simulink model "Project_Earth_Pointing"  (R2022b)
settings: Solver=VariableStepAuto  StartTime=0.0  StopTime=1000  RelTol=1e-3
values from neighbouring files (symbols this model uses):
  a = (Rp+Ra)/2    [trial_complete_project.m]    (also in trial_detumbling.m; trial_earth_pointing.m)
  A0 = Ax*Ay*Az    [trial_complete_project.m]    (also in trial_detumbling.m = [0.5391 0.1008 0.8362; -0.3591 0.9255 0.1200; -0.7618 -0.365; trial_earth_pointing.m = [-0.2505 -0.7848 0.5668; 0.7978 0.1644 0.5801; -0.5485 0.597)
  A1 = L1*L2    (= 0.06)    [trial_complete_project.m]    (also in trial_detumbling.m; trial_earth_pointing.m)
  A10 = A1    (= 0.06)    [trial_complete_project.m]    (also in trial_detumbling.m; trial_earth_pointing.m)
  A2 = A1    (= 0.06)    [trial_complete_project.m]    (also in trial_detumbling.m; trial_earth_pointing.m)
  A3 = L1*L3    (= 0.03)    [trial_complete_project.m]    (also in trial_detumbling.m; trial_earth_pointing.m)
  A4 = A3    (= 0.03)    [trial_complete_project.m]    (also in trial_detumbling.m; trial_earth_pointing.m)
  A5 = L2*L3    (= 0.02)    [trial_complete_project.m]    (also in trial_detumbling.m; trial_earth_pointing.m)
  A6 = A5    (= 0.02)    [trial_complete_project.m]    (also in trial_detumbling.m; trial_earth_pointing.m)
  A7 = A1    (= 0.06)    [trial_complete_project.m]    (also in trial_detumbling.m; trial_earth_pointing.m)
  A8 = A1    (= 0.06)    [trial_complete_project.m]    (also in trial_detumbling.m; trial_earth_pointing.m)
  A9 = A1    (= 0.06)    [trial_complete_project.m]    (also in trial_detumbling.m; trial_earth_pointing.m)
  a_s = 149600000    [trial_complete_project.m]    (also in trial_detumbling.m; trial_earth_pointing.m)
  alpha1 = 0.9    [trial_complete_project.m]    (also in trial_detumbling.m; trial_earth_pointing.m)
  alpha2 = 0.1    [trial_complete_project.m]    (also in trial_detumbling.m; trial_earth_pointing.m)
  alphaState_obs = -0.9    [trial_complete_project.m]    (also in trial_detumbling.m; trial_earth_pointing.m)
  an = (11.5*pi)/180    (= 0.200712863979)    [trial_complete_project.m]    (also in trial_detumbling.m; trial_earth_pointing.m)
  e = (Ra-Rp)/(Ra+Rp)    [trial_complete_project.m]    (also in trial_detumbling.m; trial_earth_pointing.m)
  e_s = 0.0167086    [trial_complete_project.m]    (also in trial_detumbling.m; trial_earth_pointing.m)
  i = 0*pi/180    (= 0)    [trial_complete_project.m]    (also in trial_detumbling.m; trial_earth_pointing.m)
  I_x = 0.059029338    [trial_complete_project.m]    (also in trial_detumbling.m; trial_earth_pointing.m = 0.093296)
  I_y = 0.116709338    [trial_complete_project.m]    (also in trial_detumbling.m; trial_earth_pointing.m = 0.161261916)
  I_z = 0.149968    [trial_complete_project.m]    (also in trial_detumbling.m; trial_earth_pointing.m = 0.160253916)
  kdx = kd*(I_x/I)    (= 1.44987726319)    [trial_complete_project.m]    (also in trial_detumbling.m; trial_earth_pointing.m = 2.6989394073)
  kdy = kd*(I_y/I)    (= 2.86661211697)    [trial_complete_project.m]    (also in trial_detumbling.m; trial_earth_pointing.m = 4.66511040119)
  kdz = kd*(I_z/I)    (= 3.68351061984)    [trial_complete_project.m]    (also in trial_detumbling.m; trial_earth_pointing.m = 4.63595019151)
  kpx = kp*(I_x/I)    (= 0.0163111192108)    [trial_complete_project.m]    (also in trial_detumbling.m; trial_earth_pointing.m = 0.0202420455548)
  kpy = kp*(I_y/I)    (= 0.0322493863159)    [trial_complete_project.m]    (also in trial_detumbling.m; trial_earth_pointing.m = 0.0349883280089)
  kpz = kp*(I_z/I)    (= 0.0414394944732)    [trial_complete_project.m]    (also in trial_detumbling.m; trial_earth_pointing.m = 0.0347696264363)
  kState_obs = 0.9    [trial_complete_project.m]    (also in trial_detumbling.m; trial_earth_pointing.m)
  m = [0.01 0.05 0.01]    [trial_complete_project.m]    (also in trial_detumbling.m; trial_earth_pointing.m)
  mu = astroConstants(13)    [trial_complete_project.m]    (also in trial_detumbling.m; trial_earth_pointing.m)
  n = sqrt(mu/a^3)    [trial_complete_project.m]    (also in trial_detumbling.m; trial_earth_pointing.m)
  n_s = sqrt(mu_s/a_s^3)    [trial_complete_project.m]    (also in trial_detumbling.m; trial_earth_pointing.m)
  P = F_e/c    (= 4.52980041279e-06)    [trial_complete_project.m]    (also in trial_detumbling.m; trial_earth_pointing.m)
  P_E = F_earth/c    (= 2.23487943783e-06)    [trial_complete_project.m]    (also in trial_detumbling.m; trial_earth_pointing.m)
  pd_sc = 0.1    [trial_complete_project.m]    (also in trial_detumbling.m; trial_earth_pointing.m)
  pd_sp = 0.1    [trial_complete_project.m]    (also in trial_detumbling.m; trial_earth_pointing.m)
  ps_sc = 0.5    [trial_complete_project.m]    (also in trial_detumbling.m; trial_earth_pointing.m)
  ps_sp = 0.1    [trial_complete_project.m]    (also in trial_detumbling.m; trial_earth_pointing.m)
  r = astroConstants(23)    [trial_complete_project.m]    (also in trial_detumbling.m; trial_earth_pointing.m)
  r1 = [0;0;-L3/2] + c_m    [trial_complete_project.m]    (also in trial_detumbling.m; trial_earth_pointing.m)
  r10 = r9    [trial_complete_project.m]    (also in trial_detumbling.m; trial_earth_pointing.m)
  r2 = [0; 0 ;L3/2] + c_m    [trial_complete_project.m]    (also in trial_detumbling.m; trial_earth_pointing.m)
  r3 = [0; L2/2;0] + c_m    [trial_complete_project.m]    (also in trial_detumbling.m; trial_earth_pointing.m)
  r4 = [0; -L2/2;0] + c_m    [trial_complete_project.m]    (also in trial_detumbling.m; trial_earth_pointing.m)
  r5 = [-L1/2; 0 ;0] + c_m    [trial_complete_project.m]    (also in trial_detumbling.m; trial_earth_pointing.m)
  r6 = [L1/2; 0;0]+ c_m    [trial_complete_project.m]    (also in trial_detumbling.m; trial_earth_pointing.m)
  r7 = [-L1/2; 0 ; L3/2 + L1/2] + c_m    [trial_complete_project.m]    (also in trial_detumbling.m; trial_earth_pointing.m)
  r8 = r7    [trial_complete_project.m]    (also in trial_detumbling.m; trial_earth_pointing.m)
  r9 = [-L1/2; 0 ; -L3/2 - L1/2]    [trial_complete_project.m]    (also in trial_detumbling.m; trial_earth_pointing.m)
  RW = 0.002    [trial_complete_project.m]    (also in trial_detumbling.m; trial_earth_pointing.m)
  theta0 = 0    [trial_complete_project.m]    (also in trial_detumbling.m; trial_earth_pointing.m)
  w0_x = 1    [trial_complete_project.m]    (also in trial_detumbling.m; trial_earth_pointing.m = -0.008328)
  w0_y = 1    [trial_complete_project.m]    (also in trial_detumbling.m; trial_earth_pointing.m = 0.004962)
  w0_z = 1    [trial_complete_project.m]    (also in trial_detumbling.m; trial_earth_pointing.m = -0.0004756)
  w_E = (15.04*pi/180)/3600    (= 7.29159776389e-05)    [trial_complete_project.m]    (also in trial_detumbling.m; trial_earth_pointing.m)
libraries: matrix_library x28, vrlib x7, dspinverses x1
(part 1 of 3)
settings Model: Creator=PEPPE  LastModifiedBy=PEPPE
settings SolverCC: ZeroCrossAlgorithm=Adaptive
settings DebuggingCC: IgnoredZcDiagnostic=none

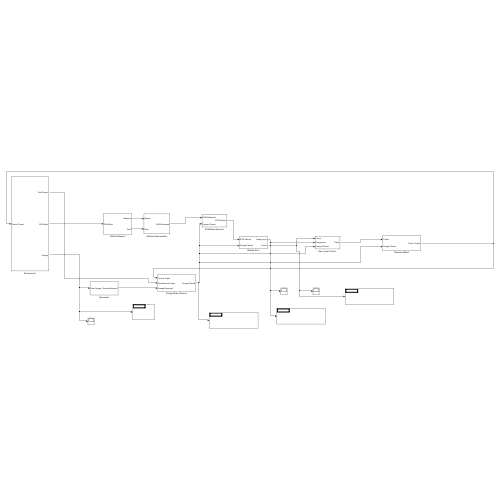
[thumbnail: Simulink's stored preview of the top-level diagram]
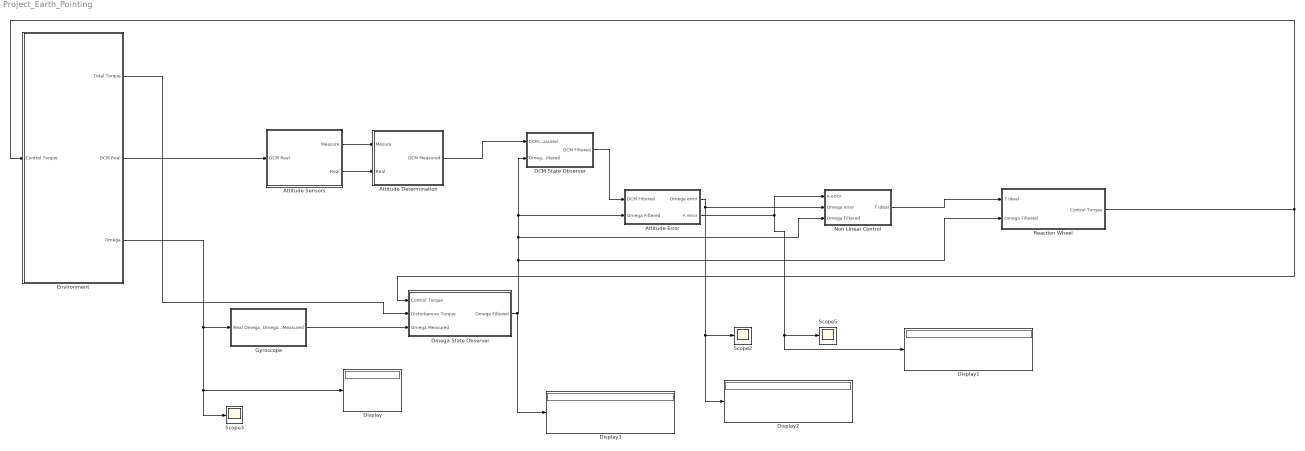
== system Project_Earth_Pointing ==
  Attitude Determination : Subsystem
  Attitude Error : Subsystem
  Attitude Sensors : Subsystem
  DCM State Observer : Subsystem
  Display{,1..3} (4 alike) : Display
  Environment : Subsystem
  Gyroscope : Subsystem
  "Non Linear Control " : Subsystem
  Omega State Observer : Subsystem
  Reaction Wheel : Subsystem
  Scope2 : Scope
  Scope3 : Scope
  Scope5 : Scope
  wires:
  Attitude Error/2(A error) -> "Non Linear Control "/1(A error), Display1/1, Scope5/1
  Environment/3(Omega) -> Display/1, Scope3/1, Gyroscope/1(Real Omega)
  Attitude Sensors/2(Real) -> Attitude Determination/2(Real)
  Environment/2(DCM Real) -> Attitude Sensors/1(DCM Real)
  Attitude Sensors/1(Measure) -> Attitude Determination/1(Mesure)
  Attitude Error/1(Omega error) -> "Non Linear Control "/2(Omega error), Display2/1, Scope2/1
  Environment/1(Total Torque) -> Omega State Observer/2(Disturbances Torque)
  Reaction Wheel/1(Control Torque) -> Environment/1(Control Torque), Omega State Observer/1(Control Torque)
  Gyroscope/1(Omega Measured) -> Omega State Observer/3(Omega Measured)
  Attitude Determination/1(DCM Measured) -> DCM State Observer/1(DCM Measured)
  Omega State Observer/1(Omega Filtered) -> Display3/1, Reaction Wheel/2(Omega Filtered), "Non Linear Control "/3(Omega Filtered), DCM State Observer/2(Omega Filtered), Attitude Error/2(Omega Filtered)
  "Non Linear Control "/1(T Ideal) -> Reaction Wheel/1(T Ideal)
  DCM State Observer/1(DCM Filtered) -> Attitude Error/1(DCM Filtered)

== system Project_Earth_Pointing/Attitude Determination ==
  Mesure : Inport
  Real : Inport  Port=2
  Demux : Demux  Outputs=2
  Demux1 : Demux  Outputs=2
  Gain : Gain  Gain=alpha1
  Gain1 : Gain  Gain=alpha2
  Gain4 : Gain  Gain=3/2
  Gain5 : Gain  Gain=1/2
  MATLAB Function : MATLAB Function  TreatAsAtomicUnit=on
  Matrix Multiply : Product  Inputs=3  Multiplication=Matrix(*)
  Matrix Multiply1 : Product  Inputs=3  Multiplication=Matrix(*)
  Matrix Multiply2 : Product  Multiplication=Matrix(*)
  Matrix Multiply3 : Product  Multiplication=Matrix(*)
  Scope : Scope
  Scope1 : Scope
  Sum : Sum  Inputs=|++
  Sum1 : Sum  Inputs=|+-
  Transpose{,1..2,5} (4 alike) : Math  Operator=transpose
  DCM Measured : Outport
  wires:
  Mesure/1 -> Demux/1
  Real/1 -> Demux1/1
  Gain/1 -> Sum/1
  Gain1/1 -> Sum/2
  Demux1/1 -> Transpose2/1
  Matrix Multiply2/1 -> Gain/1
  Demux1/2 -> Transpose5/1
  Matrix Multiply3/1 -> Gain1/1
  Demux/1 -> Matrix Multiply2/1
  Demux/2 -> Matrix Multiply3/1
  Transpose2/1 -> Matrix Multiply2/2
  Transpose5/1 -> Matrix Multiply3/2
  Gain5/1 -> Sum1/2
  Matrix Multiply/1 -> Gain4/1, Matrix Multiply1/3, Matrix Multiply1/1, Transpose/1, Scope1/1
  Transpose/1 -> Matrix Multiply1/2
  Gain4/1 -> Sum1/1
  Matrix Multiply1/1 -> Gain5/1
  Sum1/1 -> DCM Measured/1, Scope/1
  Sum/1 -> MATLAB Function/1(B)  "B"
  MATLAB Function/1(U) -> Matrix Multiply/1
  MATLAB Function/2(M) -> Matrix Multiply/2
  MATLAB Function/3(V) -> Transpose1/1
  Transpose1/1 -> Matrix Multiply/3

== system Project_Earth_Pointing/Attitude Error ==
  DCM Filtered : Inport
  Omega Filtered : Inport  Port=2
  AL_N2 : Subsystem
  Matrix Multiply : Product  Multiplication=Matrix(*)
  Matrix Multiply1 : Product  Multiplication=Matrix(*)
  Sum : Sum  Inputs=|+-
  Transpose : Math  Operator=transpose
  Vector Concatenate : Concatenate  NumInputs=3
  Zero : Constant  Value=0  OutDataTypeStr=Inherit: Inherit via back propagation
  Zero1 : Constant  Value=0  OutDataTypeStr=Inherit: Inherit via back propagation
  Zero2 : Constant  Value=n  OutDataTypeStr=Inherit: Inherit via back propagation
  Omega error : Outport
  A error : Outport  Port=2
  wires:
  Transpose/1 -> Matrix Multiply/2
  AL_N2/1(Output) -> Transpose/1
  DCM Filtered/1 -> Matrix Multiply/1
  Zero/1 -> Vector Concatenate/1
  Zero1/1 -> Vector Concatenate/2
  Zero2/1 -> Vector Concatenate/3
  Vector Concatenate/1 -> Matrix Multiply1/2
  Matrix Multiply/1 -> A error/1, Matrix Multiply1/1
  Matrix Multiply1/1 -> Sum/2
  Omega Filtered/1 -> Sum/1
  Sum/1 -> Omega error/1

== system Project_Earth_Pointing/Attitude Sensors ==
  DCM Real : Inport
  Earth Horizion Sensor : Subsystem
  Magnetometer : Subsystem
  Mux : Mux  Inputs=2
  Mux1 : Mux  Inputs=2
  Measure : Outport
  Real : Outport  Port=2
  wires:
  Mux1/1 -> Real/1
  DCM Real/1 -> Earth Horizion Sensor/1(DCM), Magnetometer/1(DCM)
  Magnetometer/1(Mesure) -> Mux/2
  Magnetometer/2(position) -> Mux1/2
  Earth Horizion Sensor/1(measure) -> Mux/1
  Earth Horizion Sensor/2(position) -> Mux1/1
  Mux/1 -> Measure/1

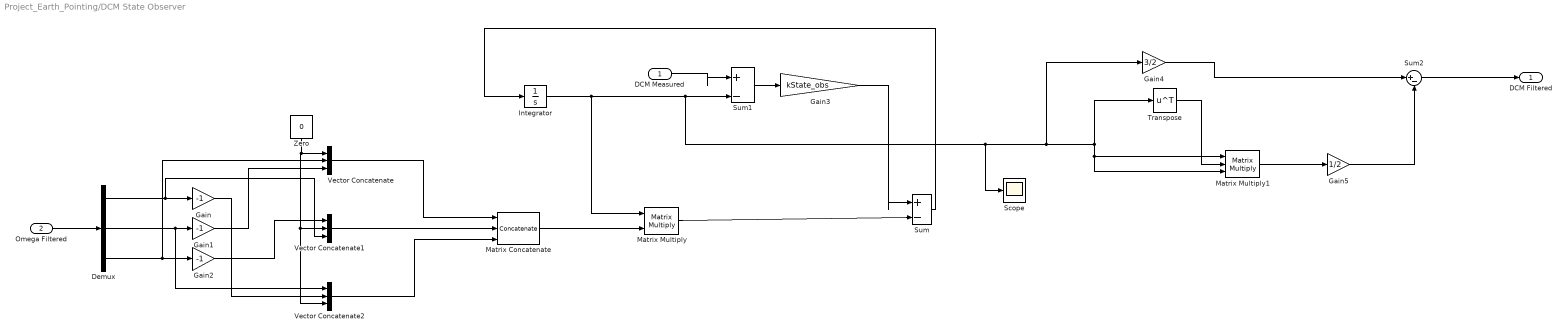
== system Project_Earth_Pointing/DCM State Observer ==
  DCM Measured : Inport
  Omega Filtered : Inport  Port=2
  Demux : Demux  Outputs=3
  Gain : Gain  Gain=-1
  Gain1 : Gain  Gain=-1
  Gain2 : Gain  Gain=-1
  Gain3 : Gain  Gain=kState_obs
  Gain4 : Gain  Gain=3/2
  Gain5 : Gain  Gain=1/2
  Integrator : Integrator  InitialCondition=A0
  Matrix Concatenate : Concatenate  NumInputs=3  Mode=Multidimensional array  ConcatenateDimension=2
  Matrix Multiply : Product  Multiplication=Matrix(*)
  Matrix Multiply1 : Product  Inputs=3  Multiplication=Matrix(*)
  Scope : Scope
  Sum : Sum  Inputs=|+-
  Sum1 : Sum  Inputs=|+-
  Sum2 : Sum  Inputs=|+-
  Transpose : Math  Operator=transpose
  Vector Concatenate : Concatenate  NumInputs=3
  Vector Concatenate1 : Concatenate  NumInputs=3
  Vector Concatenate2 : Concatenate  NumInputs=3
  Zero : Constant  Value=0  OutDataTypeStr=Inherit: Inherit via back propagation
  DCM Filtered : Outport
  wires:
  Gain5/1 -> Sum2/2
  Sum2/1 -> DCM Filtered/1
  Gain4/1 -> Sum2/1
  Matrix Multiply1/1 -> Gain5/1
  Transpose/1 -> Matrix Multiply1/2
  Integrator/1 -> Sum1/2, Transpose/1, Matrix Multiply1/1, Matrix Multiply1/3, Gain4/1, Scope/1, Matrix Multiply/1
  Sum/1 -> Integrator/1
  Gain3/1 -> Sum/1
  Sum1/1 -> Gain3/1
  DCM Measured/1 -> Sum1/1
  Matrix Multiply/1 -> Sum/2
  Matrix Concatenate/1 -> Matrix Multiply/2
  Vector Concatenate2/1 -> Matrix Concatenate/3
  Vector Concatenate/1 -> Matrix Concatenate/1
  Vector Concatenate1/1 -> Matrix Concatenate/2
  Gain/1 -> Vector Concatenate2/2
  Gain2/1 -> Vector Concatenate1/1
  Gain1/1 -> Vector Concatenate/3
  Zero/1 -> Vector Concatenate/1, Vector Concatenate1/2, Vector Concatenate2/3
  Demux/3 -> Gain2/1, Vector Concatenate/2
  Demux/2 -> Gain1/1, Vector Concatenate2/1
  Demux/1 -> Gain/1, Vector Concatenate1/3
  Omega Filtered/1 -> Demux/1

== system Project_Earth_Pointing/Environment ==
  Control Torque : Inport
  "Dynamics " : Subsystem
  ERP Torque : Subsystem
  Gravity Torque : Subsystem
  Kinematics : Subsystem
  Magnetic Torque1 : Subsystem
  SRP Torque : Subsystem
  Sum : Sum  Inputs=|+++
  Sum1 : Sum  Inputs=|++
  Total Torque : Outport
  DCM Real : Outport  Port=2
  Omega : Outport  Port=3
  wires:
  "Dynamics "/1(omega) -> Kinematics/1(omega), Omega/1
  Sum/1 -> Total Torque/1
  Gravity Torque/1(C) -> "Dynamics "/1(C)
  Gravity Torque/2(r) -> "Dynamics "/2(r)
  Gravity Torque/3(Gravity torque) -> Sum/1
  SRP Torque/1(SRP Torque) -> Sum1/1
  Control Torque/1 -> "Dynamics "/5(Control Torque)
  ERP Torque/1(ERP Torque) -> Sum1/2
  Sum1/1 -> "Dynamics "/4(SRP and ERP), Sum/3
  Kinematics/1(DCM) -> DCM Real/1, Gravity Torque/1(DCM), Magnetic Torque1/1(DCM), ERP Torque/1(DCM), SRP Torque/1(DCM)
  Magnetic Torque1/1(Magnetic Torque) -> Sum/2, "Dynamics "/3(Magnetic)

== system Project_Earth_Pointing/Gyroscope ==
  Real Omega : Inport
  Integrator : Integrator
  Random Number : RandomNumber  Variance=(0.15/sqrt(3600)*pi/180*sqrt(2000))^2  SampleTime=1/2000
  Random Number1 : RandomNumber  Variance=(0.15/sqrt(3600)*pi/180*sqrt(2000))^2  SampleTime=1/2000
  Random Number2 : RandomNumber  Variance=(0.15/sqrt(3600)*pi/180*sqrt(2000))^2  SampleTime=1/2000
  Random Number3 : RandomNumber  Variance=((0.3/3600)*(pi/180)*sqrt(2000))^2  SampleTime=1/2000
  Random Number4 : RandomNumber  Variance=((0.3/3600)*(pi/180)*sqrt(2000))^2  SampleTime=1/2000
  Random Number5 : RandomNumber  Variance=((0.3/3600)*(pi/180)*sqrt(2000))^2  SampleTime=1/2000
  Scope : Scope
  Sum : Sum  Inputs=|+++
  Vector Concatenate : Concatenate  NumInputs=3
  Vector Concatenate1 : Concatenate  NumInputs=3
  Omega Measured : Outport
  wires:
  Random Number1/1 -> Vector Concatenate/2
  Random Number/1 -> Vector Concatenate/1
  Random Number2/1 -> Vector Concatenate/3
  Random Number4/1 -> Vector Concatenate1/2
  Random Number5/1 -> Vector Concatenate1/3
  Random Number3/1 -> Vector Concatenate1/1
  Vector Concatenate1/1 -> Integrator/1  "b"
  Vector Concatenate/1 -> Sum/2  "n"
  Real Omega/1 -> Sum/1
  Sum/1 -> Omega Measured/1
  Integrator/1 -> Scope/1, Sum/3

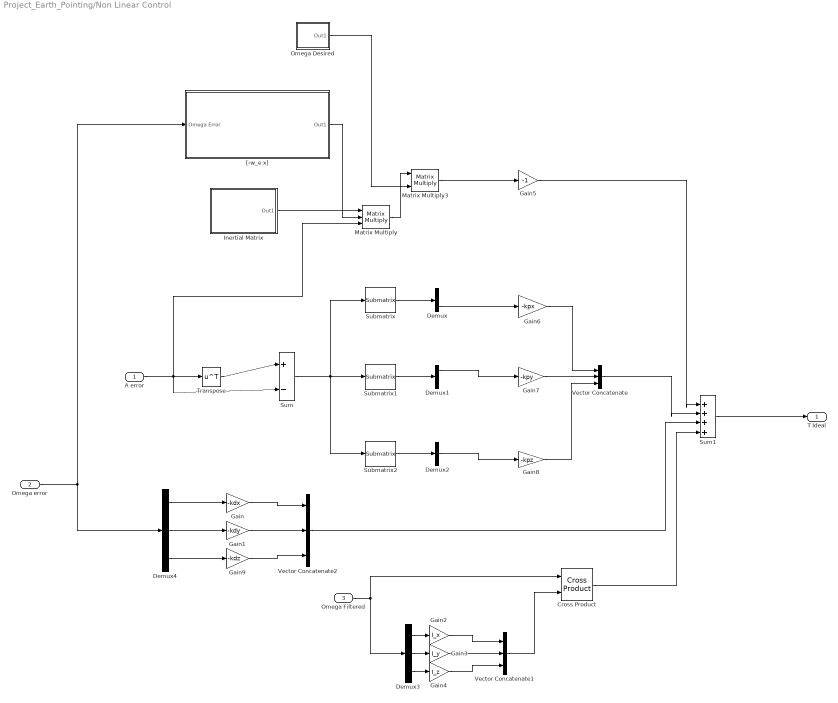
== system Project_Earth_Pointing/Non Linear Control  ==
  A error : Inport
  Omega error : Inport  Port=2
  Omega Filtered : Inport  Port=3
  Cross Product : matrix_library/Cross Product
  Demux{,1..4} (5 alike) : Demux  Outputs=3
  Gain : Gain  Gain=-kdx
  Gain1 : Gain  Gain=-kdy
  Gain2 : Gain  Gain=I_x
  Gain3 : Gain  Gain=I_y
  Gain4 : Gain  Gain=I_z
  Gain5 : Gain  Gain=-1
  Gain6 : Gain  Gain=-kpx
  Gain7 : Gain  Gain=-kpy
  Gain8 : Gain  Gain=-kpz
  Gain9 : Gain  Gain=-kdz
  Inertial Matrix : Subsystem
  Matrix Multiply : Product  Inputs=3  Multiplication=Matrix(*)
  Matrix Multiply3 : Product  Multiplication=Matrix(*)
  Omega Desired : Subsystem
  Submatrix : matrix_library/Submatrix  RowSpan=All rows  RowStartMode=First  RowStartIndex=1  RowEndMode=Last  RowEndIndex=1  ColSpan=One column  ColStartMode=Index  ColStartIndex=2  ColEndMode=Last  ColEndIndex=1
  Submatrix1 : matrix_library/Submatrix  RowSpan=All rows  RowStartMode=First  RowStartIndex=1  RowEndMode=Last  RowEndIndex=1  ColSpan=One column  ColStartMode=Last  ColStartIndex=1  ColEndMode=Last  ColEndIndex=1
  Submatrix2 : matrix_library/Submatrix  RowSpan=All rows  RowStartMode=First  RowStartIndex=1  RowEndMode=Last  RowEndIndex=1  ColSpan=One column  ColStartMode=First  ColStartIndex=1  ColEndMode=Last  ColEndIndex=1
  Sum : Sum  Inputs=|+-
  Sum1 : Sum  Inputs=|++++
  Transpose : Math  Operator=transpose
  Vector Concatenate : Concatenate  NumInputs=3
  Vector Concatenate1 : Concatenate  NumInputs=3
  Vector Concatenate2 : Concatenate  NumInputs=3
  "[-w_e x]" : Subsystem
  T Ideal : Outport
  wires:
  A error/1 -> Matrix Multiply/3, Sum/2, Transpose/1
  Transpose/1 -> Sum/1
  Omega error/1 -> Demux4/1, "[-w_e x]"/1(Omega Error)
  Sum/1 -> Submatrix2/1, Submatrix/1, Submatrix1/1
  Submatrix2/1 -> Demux2/1
  Submatrix1/1 -> Demux1/1
  Submatrix/1 -> Demux/1
  Demux/3 -> Gain6/1
  Demux1/1 -> Gain7/1
  Demux2/2 -> Gain8/1
  Vector Concatenate2/1 -> Sum1/3
  Vector Concatenate/1 -> Sum1/2
  Matrix Multiply3/1 -> Gain5/1
  Gain5/1 -> Sum1/1
  Inertial Matrix/1(Out1) -> Matrix Multiply/1
  "[-w_e x]"/1(Out1) -> Matrix Multiply/2
  Matrix Multiply/1 -> Matrix Multiply3/1
  Omega Desired/1(Out1) -> Matrix Multiply3/2
  Omega Filtered/1 -> Cross Product/1, Demux3/1
  Cross Product/1 -> Sum1/4
  Gain3/1 -> Vector Concatenate1/2
  Gain2/1 -> Vector Concatenate1/1
  Gain4/1 -> Vector Concatenate1/3
  Demux3/3 -> Gain4/1
  Demux3/2 -> Gain3/1
  Demux3/1 -> Gain2/1
  Vector Concatenate1/1 -> Cross Product/2
  Sum1/1 -> T Ideal/1
  Gain6/1 -> Vector Concatenate/1
  Gain7/1 -> Vector Concatenate/2
  Gain8/1 -> Vector Concatenate/3
  Demux4/1 -> Gain/1
  Demux4/2 -> Gain1/1
  Demux4/3 -> Gain9/1
  Gain1/1 -> Vector Concatenate2/2
  Gain/1 -> Vector Concatenate2/1
  Gain9/1 -> Vector Concatenate2/3

== system Project_Earth_Pointing/Omega State Observer ==
  Control Torque : Inport
  Disturbances Torque : Inport  Port=2
  Omega Measured : Inport  Port=3
  Cross Product : matrix_library/Cross Product
  Demux3 : Demux  Outputs=3
  Gain : Gain  Gain=alphaState_obs
  Gain3 : Gain  Gain=1/I_x
  Gain4 : Gain  Gain=1/I_y
  Gain5 : Gain  Gain=1/I_z
  Integrator : Integrator  InitialCondition=[w0_x w0_y w0_z]
  Mux : Mux  Inputs=3
  Sum : Sum  Inputs=|+++
  Sum3 : Sum  Inputs=|++
  Sum4 : Sum  Inputs=|+-
  Omega Filtered : Outport
  wires:
  Demux3/2 -> Gain4/1
  Demux3/1 -> Gain3/1
  Demux3/3 -> Gain5/1
  Gain5/1 -> Mux/3
  Disturbances Torque/1 -> Sum3/1
  Control Torque/1 -> Sum3/2
  Sum3/1 -> Demux3/1
  Omega Measured/1 -> Sum4/2
  Integrator/1 -> Cross Product/2, Cross Product/1, Sum4/1, Omega Filtered/1
  Sum4/1 -> Gain/1
  Gain3/1 -> Mux/1
  Gain4/1 -> Mux/2
  Mux/1 -> Sum/1
  Gain/1 -> Sum/2
  Cross Product/1 -> Sum/3
  Sum/1 -> Integrator/1

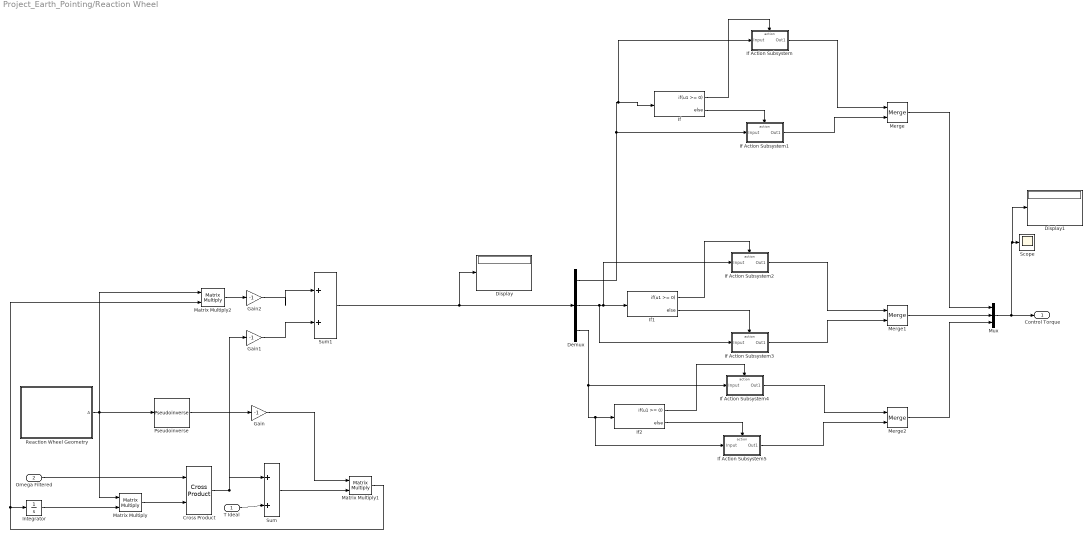
== system Project_Earth_Pointing/Reaction Wheel ==
  T Ideal : Inport
  Omega Filtered : Inport  Port=2
  Cross Product : matrix_library/Cross Product
  Demux : Demux  Outputs=3
  Display : Display
  Display1 : Display
  Gain : Gain  Gain=-1
  Gain1 : Gain  Gain=-1
  Gain2 : Gain  Gain=-1
  If : If  IfExpression=u1 >= 0
  If Action Subsystem : Subsystem  TreatAsAtomicUnit=on
  If Action Subsystem1 : Subsystem  TreatAsAtomicUnit=on
  If Action Subsystem2 : Subsystem  TreatAsAtomicUnit=on
  If Action Subsystem3 : Subsystem  TreatAsAtomicUnit=on
  If Action Subsystem4 : Subsystem  TreatAsAtomicUnit=on
  If Action Subsystem5 : Subsystem  TreatAsAtomicUnit=on
  If1 : If  IfExpression=u1 >= 0
  If2 : If  IfExpression=u1 >= 0
  Integrator : Integrator
  Matrix Multiply : Product  Multiplication=Matrix(*)
  Matrix Multiply1 : Product  Multiplication=Matrix(*)
  Matrix Multiply2 : Product  Multiplication=Matrix(*)
  Merge : Merge
  Merge1 : Merge
  Merge2 : Merge
  Mux : Mux  Inputs=3
  Pseudoinverse : dspinverses/Pseudoinverse  wanterr=off  SimulateUsing=Interpreted execution
  Reaction Wheel Geometry : Subsystem
  Scope : Scope
  Sum : Sum  Inputs=|++
  Sum1 : Sum  Inputs=|++
  Control Torque : Outport
  wires:
  If Action Subsystem5/1(Out1) -> Merge2/2
  If Action Subsystem4/1(Out1) -> Merge2/1
  If2/2 -> If Action Subsystem5/Action
  If2/1 -> If Action Subsystem4/Action
  If Action Subsystem2/1(Out1) -> Merge1/1
  If Action Subsystem3/1(Out1) -> Merge1/2
  If1/2 -> If Action Subsystem3/Action
  If1/1 -> If Action Subsystem2/Action
  If Action Subsystem/1(Out1) -> Merge/1
  If Action Subsystem1/1(Out1) -> Merge/2
  If/2 -> If Action Subsystem1/Action
  If/1 -> If Action Subsystem/Action
  Mux/1 -> Control Torque/1, Scope/1, Display1/1
  Merge2/1 -> Mux/3
  Merge1/1 -> Mux/2
  Merge/1 -> Mux/1
  Demux/3 -> If Action Subsystem4/1(Input), If2/1, If Action Subsystem5/1(Input)
  Demux/2 -> If1/1, If Action Subsystem2/1(Input), If Action Subsystem3/1(Input)
  Sum1/1 -> Demux/1, Display/1
  Gain2/1 -> Sum1/1
  Gain1/1 -> Sum1/2
  Matrix Multiply2/1 -> Gain2/1
  Matrix Multiply1/1 -> Matrix Multiply2/2, Integrator/1
  Sum/1 -> Matrix Multiply1/2
  Gain/1 -> Matrix Multiply1/1
  T Ideal/1 -> Sum/2
  Cross Product/1 -> Gain1/1, Sum/1
  Integrator/1 -> Matrix Multiply/2
  Matrix Multiply/1 -> Cross Product/2
  Omega Filtered/1 -> Cross Product/1
  Pseudoinverse/1 -> Gain/1
  Reaction Wheel Geometry/1(A) -> Matrix Multiply/1, Pseudoinverse/1, Matrix Multiply2/1
  Demux/1 -> If/1, If Action Subsystem/1(Input), If Action Subsystem1/1(Input)

== system Project_Earth_Pointing/Attitude Error/AL_N2 ==
  Clock : Clock
  Constant : Constant
  Cos : Trigonometry  Operator=cos
  Gain : Gain  Gain=n
  Gain2 : Gain  Gain=-1
  Matrix Concatenate : Concatenate  NumInputs=3  Mode=Multidimensional array  ConcatenateDimension=2
  Sin : Trigonometry
  Vector Concatenate : Concatenate  NumInputs=3
  Vector Concatenate1 : Concatenate  NumInputs=3
  Vector Concatenate2 : Concatenate  NumInputs=3
  Zero : Constant  Value=0  OutDataTypeStr=Inherit: Inherit via back propagation
  Output : Outport
  wires:
  Zero/1 -> Vector Concatenate2/1, Vector Concatenate2/2, Vector Concatenate1/3, Vector Concatenate/3
  Sin/1 -> Vector Concatenate1/1, Gain2/1
  Vector Concatenate/1 -> Matrix Concatenate/1
  Gain/1 -> Sin/1, Cos/1
  Gain2/1 -> Vector Concatenate/2
  Vector Concatenate2/1 -> Matrix Concatenate/3
  Cos/1 -> Vector Concatenate/1, Vector Concatenate1/2
  Clock/1 -> Gain/1
  Constant/1 -> Vector Concatenate2/3
  Vector Concatenate1/1 -> Matrix Concatenate/2
  Matrix Concatenate/1 -> Output/1

== system Project_Earth_Pointing/Attitude Sensors/Earth Horizion Sensor ==
  DCM : Inport
  A_epsylon : Subsystem
  Gain3 : Gain  Gain=pi/180
  Matrix Multiply : Product  Multiplication=Matrix(*)
  Matrix Multiply1 : Product  Multiplication=Matrix(*)
  Random Number : RandomNumber  Variance=0.25^2  SampleTime=0.1
  Random Number1 : RandomNumber  Variance=0.25^2  SampleTime=0.1
  Random Number2 : RandomNumber  Variance=0.25^2  SampleTime=0.1
  Theta_integration : Subsystem
  Vector Concatenate : Concatenate  NumInputs=3
  r_N : Subsystem
  measure : Outport
  position : Outport  Port=2
  wires:
  Theta_integration/1(Output) -> r_N/1(Input1)
  Gain3/1 -> A_epsylon/1(Input)
  Random Number1/1 -> Vector Concatenate/2
  Random Number/1 -> Vector Concatenate/1
  Random Number2/1 -> Vector Concatenate/3
  Vector Concatenate/1 -> Gain3/1
  DCM/1 -> Matrix Multiply/1
  r_N/1(Output) -> position/1, Matrix Multiply/2  "r_N"
  Matrix Multiply/1 -> Matrix Multiply1/2
  A_epsylon/1(Output) -> Matrix Multiply1/1
  Matrix Multiply1/1 -> measure/1

== system Project_Earth_Pointing/Attitude Sensors/Magnetometer ==
  DCM : Inport
  A_epsylon : Subsystem
  Gain1 : Gain  Gain=pi/180
  Gain3 : Gain  Gain=pi/180
  H_0 : Subsystem
  Matrix Multiply : Product  Multiplication=Matrix(*)
  Matrix Multiply1 : Product  Multiplication=Matrix(*)
  Random Number : RandomNumber  SampleTime=1/140
  Random Number1 : RandomNumber  SampleTime=1/140
  Random Number2 : RandomNumber  SampleTime=1/140
  Random Number3 : RandomNumber  Variance=(15*10^-3)^2  SampleTime=1/140
  Random Number4 : RandomNumber  Variance=(15*10^-3)^2  SampleTime=1/140
  Random Number5 : RandomNumber  Variance=(15*10^-3)^2  SampleTime=1/140
  Sum : Sum  Inputs=|++
  Theta_integration : Subsystem
  Vector Concatenate : Concatenate  NumInputs=3
  Vector Concatenate1 : Concatenate  NumInputs=3
  b_n : Subsystem
  m : Subsystem
  r_N : Subsystem
  Mesure : Outport
  position : Outport  Port=2
  wires:
  Vector Concatenate/1 -> Gain3/1
  Matrix Multiply/1 -> Mesure/1
  A_epsylon/1(Output) -> Matrix Multiply/1
  H_0/1(Output) -> b_n/2(Input)
  m/1(Output) -> b_n/3(Input3)
  r_N/1(Output) -> b_n/1(Input2)  "r_N"
  Theta_integration/1(Output) -> r_N/1(Input1)
  b_n/1(Output) -> Matrix Multiply1/2, position/1
  DCM/1 -> Matrix Multiply1/1
  Random Number/1 -> Vector Concatenate/1
  Random Number1/1 -> Vector Concatenate/2
  Random Number2/1 -> Vector Concatenate/3
  Gain3/1 -> A_epsylon/1(Input)
  Random Number5/1 -> Vector Concatenate1/3
  Vector Concatenate1/1 -> Gain1/1
  Random Number4/1 -> Vector Concatenate1/2
  Random Number3/1 -> Vector Concatenate1/1
  Matrix Multiply1/1 -> Sum/1  "b_b"
  Gain1/1 -> Sum/2
  Sum/1 -> Matrix Multiply/2

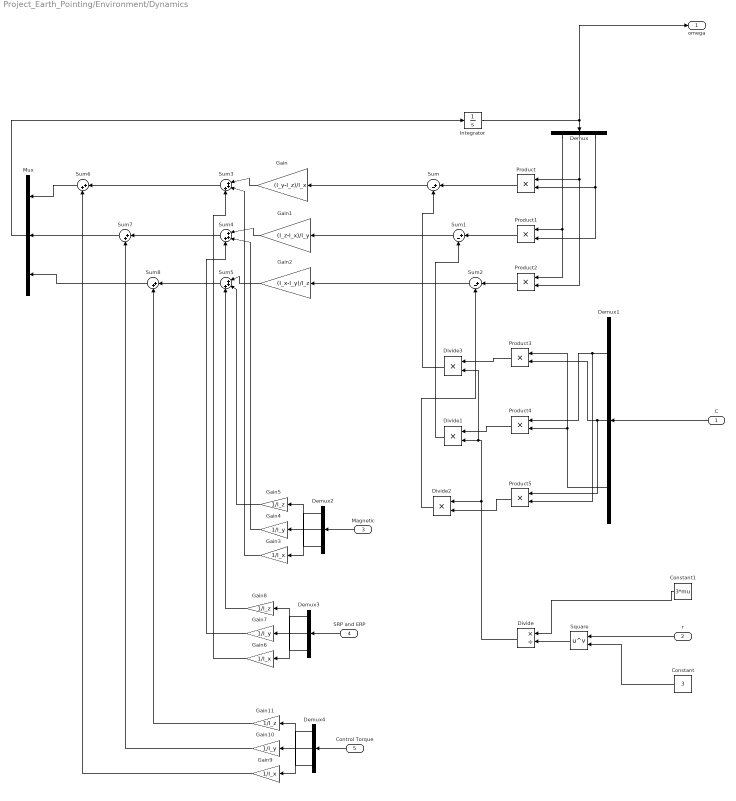
== system Project_Earth_Pointing/Environment/Dynamics  ==
  C : Inport
  r : Inport  Port=2
  Magnetic : Inport  Port=3
  SRP and ERP : Inport  Port=4
  Control Torque : Inport  Port=5
  Constant : Constant  Value=3
  Constant1 : Constant  Value=3*mu
  Demux{,1..4} (5 alike) : Demux  Outputs=3
  Divide : Product  Inputs=*/  RndMeth=Zero  SaturateOnIntegerOverflow=on
  Divide1 : Product  Inputs=**  RndMeth=Zero  SaturateOnIntegerOverflow=on
  Divide2 : Product  Inputs=**  RndMeth=Zero  SaturateOnIntegerOverflow=on
  Divide3 : Product  Inputs=**  RndMeth=Zero  SaturateOnIntegerOverflow=on
  Gain : Gain  Gain=(I_y-I_z)/I_x
  Gain1 : Gain  Gain=(I_z-I_x)/I_y
  Gain10 : Gain  Gain=1/I_y
  Gain11 : Gain  Gain=1/I_z
  Gain2 : Gain  Gain=(I_x-I_y)/I_z
  Gain3 : Gain  Gain=1/I_x
  Gain4 : Gain  Gain=1/I_y
  Gain5 : Gain  Gain=1/I_z
  Gain6 : Gain  Gain=1/I_x
  Gain7 : Gain  Gain=1/I_y
  Gain8 : Gain  Gain=1/I_z
  Gain9 : Gain  Gain=1/I_x
  Integrator : Integrator  InitialCondition=[w0_x w0_y w0_z]
  Mux : Mux  Inputs=3
  Product{,1..5} (6 alike) : Product
  Square : Math  Operator=pow
  Sum : Sum  Inputs=|+-
  Sum1 : Sum  Inputs=|+-
  Sum2 : Sum  Inputs=|+-
  Sum3 : Sum  Inputs=|+++
  Sum4 : Sum  Inputs=|+++
  Sum5 : Sum  Inputs=|+++
  Sum6 : Sum  Inputs=|++
  Sum7 : Sum  Inputs=|++
  Sum8 : Sum  Inputs=|++
  omega : Outport
  wires:
  Demux/2 -> Product2/2, Product/1
  Demux/1 -> Product2/1, Product1/1
  Integrator/1 -> omega/1, Demux/1
  Demux/3 -> Product1/2, Product/2
  Product/1 -> Sum/1
  Product1/1 -> Sum1/1
  Product2/1 -> Sum2/1
  Sum/1 -> Gain/1
  Sum1/1 -> Gain1/1
  Sum2/1 -> Gain2/1
  C/1 -> Demux1/1
  Demux1/3 -> Product4/2, Product3/1
  Demux1/2 -> Product5/1, Product3/2
  Demux1/1 -> Product5/2, Product4/1
  Divide3/1 -> Sum/2
  Divide1/1 -> Sum1/2
  Divide2/1 -> Sum2/2
  Mux/1 -> Integrator/1
  r/1 -> Square/1
  Constant/1 -> Square/2
  Constant1/1 -> Divide/1
  Square/1 -> Divide/2
  Divide/1 -> Divide3/2, Divide1/2, Divide2/1
  Product5/1 -> Divide2/2
  Product4/1 -> Divide1/1
  Product3/1 -> Divide3/1
  Demux2/2 -> Gain4/1
  Magnetic/1 -> Demux2/1
  Demux2/3 -> Gain5/1
  Demux2/1 -> Gain3/1
  Gain2/1 -> Sum5/1
  Gain1/1 -> Sum4/1
  Gain/1 -> Sum3/1
  Gain3/1 -> Sum3/2
  Gain4/1 -> Sum4/2
  Gain5/1 -> Sum5/2
  SRP and ERP/1 -> Demux3/1
  Demux3/3 -> Gain8/1
  Demux3/2 -> Gain7/1
  Demux3/1 -> Gain6/1
  Gain8/1 -> Sum5/3
  Gain7/1 -> Sum4/3
  Gain6/1 -> Sum3/3
  Demux4/2 -> Gain10/1
  Demux4/1 -> Gain9/1
  Control Torque/1 -> Demux4/1
  Demux4/3 -> Gain11/1
  Sum3/1 -> Sum6/1
  Sum4/1 -> Sum7/1
  Sum5/1 -> Sum8/1
  Gain11/1 -> Sum8/2
  Gain10/1 -> Sum7/2
  Gain9/1 -> Sum6/2
  Sum6/1 -> Mux/1
  Sum7/1 -> Mux/2
  Sum8/1 -> Mux/3

== system Project_Earth_Pointing/Environment/ERP Torque ==
  note: n (for the earth)
      | e (sc orbit)
      | i (sc orbit)
      | a (sc orbit)
      | P_E (F_E from earth radiation)
      | A (surface areas 1-10)
      | rho_s and rho_d
  note: list of initial conditions needed:
  DCM : Inport
  Matrix Multiply3 : Product  Multiplication=Matrix(*)
  Mux : Mux  Inputs=10
  Mux1 : Mux  Inputs=10
  Spacecraft Geometry : Subsystem
  Subsystem : Subsystem
  Subsystem10 : Subsystem
  Subsystem11 : Subsystem
  Subsystem2 : Subsystem
  Subsystem3 : Subsystem
  Subsystem4 : Subsystem
  Subsystem5 : Subsystem
  Subsystem6 : Subsystem
  Subsystem7 : Subsystem
  Subsystem8 : Subsystem
  Subsystem9 : Subsystem
  Theta_integration : Subsystem
  r_n : Subsystem
  ERP Torque : Outport
  wires:
  Subsystem11/1(Output) -> ERP Torque/1
  Subsystem4/2(Output1) -> Mux/4
  Subsystem8/2(Output1) -> Mux/8
  Subsystem9/2(Output1) -> Mux/9
  Subsystem2/1(Output) -> Mux1/2
  Subsystem5/1(Output) -> Mux1/5
  Mux/1 -> Subsystem11/2(Input1)
  Spacecraft Geometry/10(Output9) -> Subsystem10/2(Input1)
  Spacecraft Geometry/1(Output) -> Subsystem/2(Input1)
  Spacecraft Geometry/9(Output8) -> Subsystem9/2(Input1)
  Subsystem10/2(Output1) -> Mux/10
  Subsystem7/2(Output1) -> Mux/7
  r_n/1(Output) -> Matrix Multiply3/2
  Subsystem3/1(Output) -> Mux1/3
  Spacecraft Geometry/5(Output4) -> Subsystem5/2(Input1)
  DCM/1 -> Matrix Multiply3/1
  Spacecraft Geometry/3(Output2) -> Subsystem3/2(Input1)
  Subsystem3/2(Output1) -> Mux/3
  Mux1/1 -> Subsystem11/1(Input)
  Subsystem10/1(Output) -> Mux1/10
  Spacecraft Geometry/8(Output7) -> Subsystem8/2(Input1)
  Subsystem2/2(Output1) -> Mux/2
  Spacecraft Geometry/7(Output6) -> Subsystem7/2(Input1)
  Subsystem/2(Output1) -> Mux/1
  Subsystem/1(Output) -> Mux1/1
  Matrix Multiply3/1 -> Subsystem/1(Input), Subsystem2/1(Input), Subsystem3/1(Input), Subsystem4/1(Input), Subsystem5/1(Input), Subsystem6/1(Input), Subsystem7/1(Input), Subsystem8/1(Input), Subsystem9/1(Input), Subsystem10/1(Input)
  Subsystem5/2(Output1) -> Mux/5
  Subsystem8/1(Output) -> Mux1/8
  Subsystem4/1(Output) -> Mux1/4
  Theta_integration/1(Output) -> r_n/1(theta)
  Subsystem6/2(Output1) -> Mux/6
  Subsystem7/1(Output) -> Mux1/7
  Subsystem9/1(Output) -> Mux1/9
  Subsystem6/1(Output) -> Mux1/6
  Spacecraft Geometry/6(Output5) -> Subsystem6/2(Input1)
  Spacecraft Geometry/4(Output3) -> Subsystem4/2(Input1)
  Spacecraft Geometry/2(Output1) -> Subsystem2/2(Input1)

== system Project_Earth_Pointing/Environment/Gravity Torque ==
  DCM : Inport
  A_L_N : Subsystem
  Constant : Constant  Value=0
  Matrix Multiply : Product  Multiplication=Matrix(*)
  Matrix Multiply1 : Product  Multiplication=Matrix(*)
  Transpose : Math  Operator=transpose
  Two_body_problem : Subsystem
  Vector Concatenate : Concatenate  NumInputs=3
  Zero : Constant  OutDataTypeStr=Inherit: Inherit via back propagation
  Zero1 : Constant  Value=0  OutDataTypeStr=Inherit: Inherit via back propagation
  grav_torque : Subsystem
  C : Outport
  r : Outport  Port=2
  Gravity torque : Outport  Port=3
  wires:
  Matrix Multiply/1 -> Matrix Multiply1/1
  Two_body_problem/2(theta) -> A_L_N/1(theta)
  Matrix Multiply1/1 -> grav_torque/1(Input), C/1
  A_L_N/1(A_L_N) -> Transpose/1
  Zero/1 -> Vector Concatenate/1
  Transpose/1 -> Matrix Multiply/2
  Constant/1 -> Vector Concatenate/3
  Two_body_problem/1(r) -> r/1, grav_torque/2(Input1)
  Vector Concatenate/1 -> Matrix Multiply1/2
  DCM/1 -> Matrix Multiply/1
  Zero1/1 -> Vector Concatenate/2
  grav_torque/1(Output) -> Gravity torque/1

== system Project_Earth_Pointing/Environment/Kinematics ==
  omega : Inport
  Constant : Constant  Value=0
  Constant1 : Constant  Value=0
  Constant2 : Constant  Value=0
  Demux : Demux  Outputs=3
  Gain{,1..3} (4 alike) : Gain  Gain=-1
  Gain4 : Gain  Gain=3/2
  Gain5 : Gain  Gain=1/2
  Integrator : Integrator  InitialCondition=A0
  Matrix Concatenate : Concatenate  NumInputs=3  Mode=Multidimensional array  ConcatenateDimension=2
  Matrix Multiply : Product  Multiplication=Matrix(*)
  Matrix Multiply1 : Product  Inputs=3  Multiplication=Matrix(*)
  Sum : Sum  Inputs=|+-
  Transpose : Math  Operator=transpose
  Vector Concatenate : Concatenate  NumInputs=3
  Vector Concatenate1 : Concatenate  NumInputs=3
  Vector Concatenate2 : Concatenate  NumInputs=3
  DCM : Outport
  wires:
  Demux/2 -> Vector Concatenate2/1, Gain/1
  Gain1/1 -> Vector Concatenate1/1
  Integrator/1 -> Matrix Multiply/2, Gain4/1, Matrix Multiply1/3, Matrix Multiply1/1, Transpose/1
  Vector Concatenate2/1 -> Matrix Concatenate/3
  Gain5/1 -> Sum/2
  Vector Concatenate1/1 -> Matrix Concatenate/2
  Constant2/1 -> Vector Concatenate2/3
  Demux/3 -> Gain1/1, Vector Concatenate/2
  Transpose/1 -> Matrix Multiply1/2
  Constant1/1 -> Vector Concatenate1/2
  Demux/1 -> Gain2/1, Vector Concatenate1/3
  Matrix Multiply/1 -> Integrator/1
  Gain/1 -> Vector Concatenate/3
  Constant/1 -> Vector Concatenate/1
  Gain4/1 -> Sum/1
  omega/1 -> Demux/1
  Gain2/1 -> Vector Concatenate2/2
  Matrix Concatenate/1 -> Gain3/1
  Vector Concatenate/1 -> Matrix Concatenate/1
  Matrix Multiply1/1 -> Gain5/1
  Sum/1 -> DCM/1
  Gain3/1 -> Matrix Multiply/1

== system Project_Earth_Pointing/Environment/Magnetic Torque1 ==
  DCM : Inport
  Constant1 : Constant  Value=m
  Cross Product : matrix_library/Cross Product
  H_0 : Subsystem
  Matrix Multiply2 : Product  Multiplication=Matrix(*)
  Scope : Scope
  Theta_integration : Subsystem
  b_n : Subsystem
  m : Subsystem
  r_N : Subsystem
  Magnetic Torque : Outport
  wires:
  b_n/1(Output) -> Scope/1, Matrix Multiply2/2
  Matrix Multiply2/1 -> Cross Product/2
  Cross Product/1 -> Magnetic Torque/1
  H_0/1(Output) -> b_n/2(Input)
  r_N/1(Output) -> b_n/1(Input2)  "r_N"
  Constant1/1 -> Cross Product/1
  DCM/1 -> Matrix Multiply2/1
  m/1(Output) -> b_n/3(Input3)
  Theta_integration/1(Output) -> r_N/1(Input1)

== system Project_Earth_Pointing/Environment/SRP Torque ==
  DCM : Inport
  Matrix Multiply3 : Product  Multiplication=Matrix(*)
  Mux : Mux  Inputs=10
  Mux1 : Mux  Inputs=10
  S_n : Subsystem
  Spacecraft Geometry : Subsystem
  Subsystem : Subsystem
  Subsystem10 : Subsystem
  Subsystem11 : Subsystem
  Subsystem2 : Subsystem
  Subsystem3 : Subsystem
  Subsystem4 : Subsystem
  Subsystem5 : Subsystem
  Subsystem6 : Subsystem
  Subsystem7 : Subsystem
  Subsystem8 : Subsystem
  Subsystem9 : Subsystem
  Theta_integration : Subsystem
  SRP Torque : Outport
  wires:
  Spacecraft Geometry/2(Output1) -> Subsystem2/2(Input1)
  Spacecraft Geometry/4(Output3) -> Subsystem4/2(Input1)
  Spacecraft Geometry/6(Output5) -> Subsystem6/2(Input1)
  Subsystem6/1(Output) -> Mux1/6
  Subsystem9/1(Output) -> Mux1/9
  Subsystem7/1(Output) -> Mux1/7
  Subsystem6/2(Output1) -> Mux/6
  Theta_integration/1(Output) -> S_n/1(Input)
  Subsystem4/1(Output) -> Mux1/4
  Subsystem8/1(Output) -> Mux1/8
  Subsystem5/2(Output1) -> Mux/5
  Matrix Multiply3/1 -> Subsystem10/1(Input), Subsystem9/1(Input), Subsystem8/1(Input), Subsystem7/1(Input), Subsystem6/1(Input), Subsystem5/1(Input), Subsystem4/1(Input), Subsystem3/1(Input), Subsystem2/1(Input), Subsystem/1(Input)
  Subsystem/1(Output) -> Mux1/1
  Subsystem/2(Output1) -> Mux/1
  Spacecraft Geometry/7(Output6) -> Subsystem7/2(Input1)
  Subsystem2/2(Output1) -> Mux/2
  Spacecraft Geometry/8(Output7) -> Subsystem8/2(Input1)
  Subsystem10/1(Output) -> Mux1/10
  Mux1/1 -> Subsystem11/1(Input)
  Subsystem3/2(Output1) -> Mux/3
  Spacecraft Geometry/3(Output2) -> Subsystem3/2(Input1)
  DCM/1 -> Matrix Multiply3/1
  Spacecraft Geometry/5(Output4) -> Subsystem5/2(Input1)
  Subsystem3/1(Output) -> Mux1/3
  S_n/1(Output) -> Matrix Multiply3/2
  Subsystem7/2(Output1) -> Mux/7
  Subsystem10/2(Output1) -> Mux/10
  Spacecraft Geometry/9(Output8) -> Subsystem9/2(Input1)
  Spacecraft Geometry/1(Output) -> Subsystem/2(Input1)
  Spacecraft Geometry/10(Output9) -> Subsystem10/2(Input1)
  Mux/1 -> Subsystem11/2(Input1)
  Subsystem5/1(Output) -> Mux1/5
  Subsystem2/1(Output) -> Mux1/2
  Subsystem9/2(Output1) -> Mux/9
  Subsystem8/2(Output1) -> Mux/8
  Subsystem4/2(Output1) -> Mux/4
  Subsystem11/1(Output) -> SRP Torque/1

== system Project_Earth_Pointing/Non Linear Control /Inertial Matrix ==
  Constant : Constant  Value=I_x
  Constant1 : Constant  Value=I_y
  Constant2 : Constant  Value=I_z
  Create Diagonal Matrix : matrix_library/Create Diagonal Matrix
      settings: LibrarySourceBlock=|
      | simulink/Matrix
      | Operations/Create Diagonal
      | Matrix
  Vector Concatenate : Concatenate  NumInputs=3
  Out1 : Outport
  wires:
  Create Diagonal Matrix/1 -> Out1/1
  Constant1/1 -> Vector Concatenate/2
  Constant/1 -> Vector Concatenate/1
  Constant2/1 -> Vector Concatenate/3
  Vector Concatenate/1 -> Create Diagonal Matrix/1

== system Project_Earth_Pointing/Non Linear Control /Omega Desired ==
  Constant : Constant  Value=0
  Constant1 : Constant  Value=0
  Constant2 : Constant  Value=n
  Vector Concatenate : Concatenate  NumInputs=3
  Out1 : Outport
  wires:
  Constant1/1 -> Vector Concatenate/2
  Constant/1 -> Vector Concatenate/1
  Constant2/1 -> Vector Concatenate/3
  Vector Concatenate/1 -> Out1/1

== system Project_Earth_Pointing/Non Linear Control /[-w_e x] ==
  Omega Error : Inport
  Demux : Demux  Outputs=3
  Gain : Gain  Gain=-1
  Gain1 : Gain  Gain=-1
  Gain2 : Gain  Gain=-1
  Matrix Concatenate : Concatenate  NumInputs=3  Mode=Multidimensional array  ConcatenateDimension=2
  Vector Concatenate : Concatenate  NumInputs=3
  Vector Concatenate1 : Concatenate  NumInputs=3
  Vector Concatenate2 : Concatenate  NumInputs=3
  Zero : Constant  Value=0  OutDataTypeStr=Inherit: Inherit via back propagation
  Out1 : Outport
  wires:
  Vector Concatenate2/1 -> Matrix Concatenate/3
  Gain/1 -> Vector Concatenate2/2
  Vector Concatenate1/1 -> Matrix Concatenate/2
  Vector Concatenate/1 -> Matrix Concatenate/1
  Gain1/1 -> Vector Concatenate/3
  Zero/1 -> Vector Concatenate2/3, Vector Concatenate1/2, Vector Concatenate/1
  Omega Error/1 -> Demux/1
  Gain2/1 -> Vector Concatenate1/1
  Demux/2 -> Vector Concatenate2/1, Gain1/1
  Demux/1 -> Vector Concatenate1/3, Gain/1
  Demux/3 -> Vector Concatenate/2, Gain2/1
  Matrix Concatenate/1 -> Out1/1

== system Project_Earth_Pointing/Reaction Wheel/If Action Subsystem ==
  Input : Inport
  Action Port : ActionPort  ActionPortLabel=if(u1 >= 0)
  If : If  IfExpression=u1 <RWmin  ElseIfExpressions=u1>=RW
  If Action Subsystem : Subsystem  TreatAsAtomicUnit=on
  If Action Subsystem1 : Subsystem  TreatAsAtomicUnit=on
  If Action Subsystem2 : Subsystem  TreatAsAtomicUnit=on
  Merge : Merge  Inputs=3
  Out1 : Outport
  wires:
  Merge/1 -> Out1/1
  If Action Subsystem2/1(Out1) -> Merge/3
  If Action Subsystem/1(Out1) -> Merge/1
  If Action Subsystem1/1(Out1) -> Merge/2
  If/3 -> If Action Subsystem2/Action
  If/2 -> If Action Subsystem1/Action
  If/1 -> If Action Subsystem/Action
  Input/1 -> If/1, If Action Subsystem2/1(Input)

== system Project_Earth_Pointing/Reaction Wheel/If Action Subsystem1 ==
  Input : Inport
  Action Port : ActionPort  ActionPortLabel=else
  If : If  IfExpression=u1 >-RWmin  ElseIfExpressions=u1<=-RW
  If Action Subsystem : Subsystem  TreatAsAtomicUnit=on
  If Action Subsystem1 : Subsystem  TreatAsAtomicUnit=on
  If Action Subsystem2 : Subsystem  TreatAsAtomicUnit=on
  Merge : Merge  Inputs=3
  Out1 : Outport
  wires:
  Input/1 -> If Action Subsystem2/1(Input), If/1
  If/1 -> If Action Subsystem/Action
  If/2 -> If Action Subsystem1/Action
  If/3 -> If Action Subsystem2/Action
  If Action Subsystem1/1(Out1) -> Merge/2
  If Action Subsystem/1(Out1) -> Merge/1
  If Action Subsystem2/1(Out1) -> Merge/3
  Merge/1 -> Out1/1

== system Project_Earth_Pointing/Reaction Wheel/If Action Subsystem2 ==
  Input : Inport
  Action Port : ActionPort  ActionPortLabel=if(u1 >= 0)
  If : If  IfExpression=u1 <RWmin  ElseIfExpressions=u1>=RW
  If Action Subsystem : Subsystem  TreatAsAtomicUnit=on
  If Action Subsystem1 : Subsystem  TreatAsAtomicUnit=on
  If Action Subsystem2 : Subsystem  TreatAsAtomicUnit=on
  Merge : Merge  Inputs=3
  Out1 : Outport
  wires:
  Input/1 -> If Action Subsystem2/1(Input), If/1
  If/1 -> If Action Subsystem/Action
  If/2 -> If Action Subsystem1/Action
  If/3 -> If Action Subsystem2/Action
  If Action Subsystem1/1(Out1) -> Merge/2
  If Action Subsystem/1(Out1) -> Merge/1
  If Action Subsystem2/1(Out1) -> Merge/3
  Merge/1 -> Out1/1

== system Project_Earth_Pointing/Reaction Wheel/If Action Subsystem3 ==
  Input : Inport
  Action Port : ActionPort  ActionPortLabel=else
  If : If  IfExpression=u1 >-RWmin  ElseIfExpressions=u1<=-RW
  If Action Subsystem : Subsystem  TreatAsAtomicUnit=on
  If Action Subsystem1 : Subsystem  TreatAsAtomicUnit=on
  If Action Subsystem2 : Subsystem  TreatAsAtomicUnit=on
  Merge : Merge  Inputs=3
  Out1 : Outport
  wires:
  Merge/1 -> Out1/1
  If Action Subsystem2/1(Out1) -> Merge/3
  If Action Subsystem/1(Out1) -> Merge/1
  If Action Subsystem1/1(Out1) -> Merge/2
  If/3 -> If Action Subsystem2/Action
  If/2 -> If Action Subsystem1/Action
  If/1 -> If Action Subsystem/Action
  Input/1 -> If/1, If Action Subsystem2/1(Input)

== system Project_Earth_Pointing/Reaction Wheel/If Action Subsystem4 ==
  Input : Inport
  Action Port : ActionPort  ActionPortLabel=if(u1 >= 0)
  If : If  IfExpression=u1 <RWmin  ElseIfExpressions=u1>=RW
  If Action Subsystem : Subsystem  TreatAsAtomicUnit=on
  If Action Subsystem1 : Subsystem  TreatAsAtomicUnit=on
  If Action Subsystem2 : Subsystem  TreatAsAtomicUnit=on
  Merge : Merge  Inputs=3
  Out1 : Outport
  wires:
  Merge/1 -> Out1/1
  If Action Subsystem2/1(Out1) -> Merge/3
  If Action Subsystem/1(Out1) -> Merge/1
  If Action Subsystem1/1(Out1) -> Merge/2
  If/3 -> If Action Subsystem2/Action
  If/2 -> If Action Subsystem1/Action
  If/1 -> If Action Subsystem/Action
  Input/1 -> If/1, If Action Subsystem2/1(Input)

== system Project_Earth_Pointing/Reaction Wheel/If Action Subsystem5 ==
  Input : Inport
  Action Port : ActionPort  ActionPortLabel=else
  If : If  IfExpression=u1 >-RWmin  ElseIfExpressions=u1<=-RW
  If Action Subsystem : Subsystem  TreatAsAtomicUnit=on
  If Action Subsystem1 : Subsystem  TreatAsAtomicUnit=on
  If Action Subsystem2 : Subsystem  TreatAsAtomicUnit=on
  Merge : Merge  Inputs=3
  Out1 : Outport
  wires:
  Input/1 -> If Action Subsystem2/1(Input), If/1
  If/1 -> If Action Subsystem/Action
  If/2 -> If Action Subsystem1/Action
  If/3 -> If Action Subsystem2/Action
  If Action Subsystem1/1(Out1) -> Merge/2
  If Action Subsystem/1(Out1) -> Merge/1
  If Action Subsystem2/1(Out1) -> Merge/3
  Merge/1 -> Out1/1

== system Project_Earth_Pointing/Reaction Wheel/Reaction Wheel Geometry ==
  Constant : Constant  Value=1/sqrt(3)
  Gain : Gain  Gain=-1
  Matrix Concatenate : Concatenate  NumInputs=4  Mode=Multidimensional array  ConcatenateDimension=2
  Vector Concatenate{,1..3} (4 alike) : Concatenate  NumInputs=3
  A : Outport
  wires:
  Matrix Concatenate/1 -> A/1
  Vector Concatenate3/1 -> Matrix Concatenate/4
  Vector Concatenate2/1 -> Matrix Concatenate/3
  Vector Concatenate1/1 -> Matrix Concatenate/2
  Vector Concatenate/1 -> Matrix Concatenate/1
  Gain/1 -> Vector Concatenate/1, Vector Concatenate/2, Vector Concatenate1/2, Vector Concatenate3/1
  Constant/1 -> Gain/1, Vector Concatenate2/1, Vector Concatenate2/2, Vector Concatenate2/3, Vector Concatenate3/2, Vector Concatenate3/3, Vector Concatenate1/3, Vector Concatenate1/1, Vector Concatenate/3

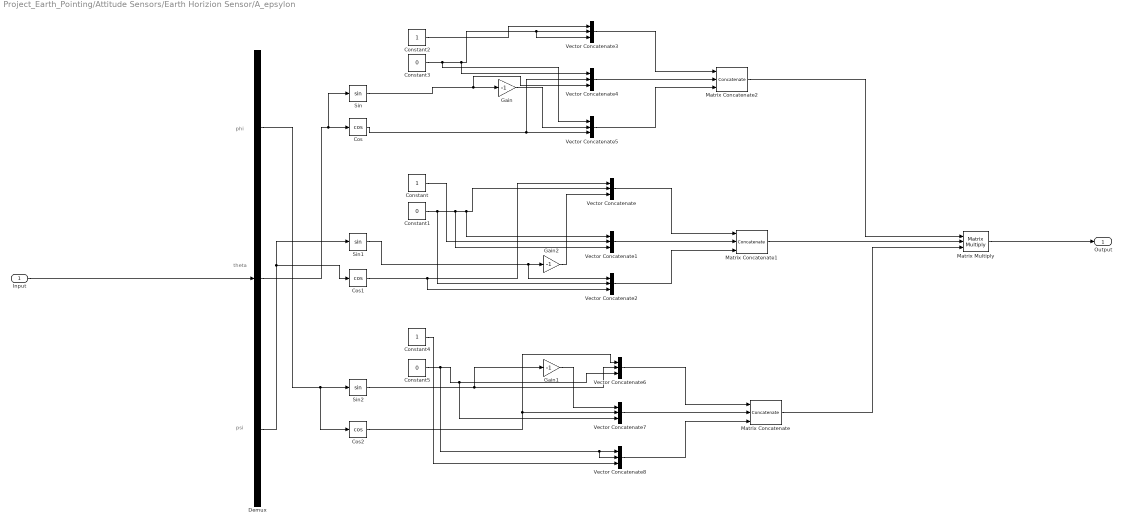
== system Project_Earth_Pointing/Attitude Sensors/Earth Horizion Sensor/A_epsylon ==
  note: phi
  note: psi
  note: theta
  Input : Inport
  Constant : Constant
  Constant1 : Constant  Value=0
  Constant2 : Constant
  Constant3 : Constant  Value=0
  Constant4 : Constant
  Constant5 : Constant  Value=0
  Cos : Trigonometry  Operator=cos
  Cos1 : Trigonometry  Operator=cos
  Cos2 : Trigonometry  Operator=cos
  Demux : Demux  Outputs=3
  Gain : Gain  Gain=-1
  Gain1 : Gain  Gain=-1
  Gain2 : Gain  Gain=-1
  Matrix Concatenate : Concatenate  NumInputs=3  Mode=Multidimensional array  ConcatenateDimension=2
  Matrix Concatenate1 : Concatenate  NumInputs=3  Mode=Multidimensional array  ConcatenateDimension=2
  Matrix Concatenate2 : Concatenate  NumInputs=3  Mode=Multidimensional array  ConcatenateDimension=2
  Matrix Multiply : Product  Inputs=3  Multiplication=Matrix(*)
  Sin : Trigonometry
  Sin1 : Trigonometry
  Sin2 : Trigonometry
  Vector Concatenate{,1..8} (9 alike) : Concatenate  NumInputs=3
  Output : Outport
  wires:
  Sin2/1 -> Vector Concatenate6/2, Gain1/1
  Sin1/1 -> Vector Concatenate2/1, Gain2/1
  Input/1 -> Demux/1
  Matrix Concatenate2/1 -> Matrix Multiply/1
  Constant5/1 -> Vector Concatenate8/2, Vector Concatenate8/1, Vector Concatenate7/3, Vector Concatenate6/3
  Matrix Multiply/1 -> Output/1
  Matrix Concatenate1/1 -> Matrix Multiply/2
  Constant3/1 -> Vector Concatenate5/1, Vector Concatenate4/1, Vector Concatenate3/3, Vector Concatenate3/2
  Sin/1 -> Vector Concatenate4/3, Gain/1
  Cos1/1 -> Vector Concatenate2/3, Vector Concatenate/1
  Vector Concatenate8/1 -> Matrix Concatenate/3
  Constant1/1 -> Vector Concatenate2/2, Vector Concatenate1/3, Vector Concatenate1/1, Vector Concatenate/2
  Demux/3 -> Sin1/1, Cos1/1
  Demux/1 -> Cos2/1, Sin2/1
  Vector Concatenate3/1 -> Matrix Concatenate2/1
  Demux/2 -> Sin/1, Cos/1
  Cos/1 -> Vector Concatenate5/3, Vector Concatenate4/2
  Constant4/1 -> Vector Concatenate8/3
  Vector Concatenate5/1 -> Matrix Concatenate2/3
  Vector Concatenate4/1 -> Matrix Concatenate2/2
  Vector Concatenate/1 -> Matrix Concatenate1/1
  Gain2/1 -> Vector Concatenate/3
  Vector Concatenate7/1 -> Matrix Concatenate/2
  Cos2/1 -> Vector Concatenate7/2, Vector Concatenate6/1
  Constant2/1 -> Vector Concatenate3/1
  Vector Concatenate1/1 -> Matrix Concatenate1/2
  Constant/1 -> Vector Concatenate1/2
  Matrix Concatenate/1 -> Matrix Multiply/3
  Vector Concatenate6/1 -> Matrix Concatenate/1
  Vector Concatenate2/1 -> Matrix Concatenate1/3
  Gain/1 -> Vector Concatenate5/2
  Gain1/1 -> Vector Concatenate7/1

== system Project_Earth_Pointing/Attitude Sensors/Earth Horizion Sensor/Theta_integration ==
  Constant : Constant
  Constant1 : Constant  Value=e
  Constant2 : Constant  Value=e
  Constant3 : Constant
  Constant4 : Constant  Value=3/2
  Cos : Trigonometry  Operator=cos
  Divide : Product  Inputs=*/
  Gain : Gain  Gain=n
  Integrator : Integrator  InitialCondition=theta0
  Product : Product
  Scope : Scope
  Scope1 : Scope
  Square : Math  Operator=square
  Square1 : Math  Operator=square
  Square2 : Math  Operator=pow
  Sum : Sum  Inputs=|++
  Sum1 : Sum  Inputs=|+-
  Output : Outport
  wires:
  Constant1/1 -> Product/1
  Integrator/1 -> Output/1, Scope/1, Cos/1
  Constant3/1 -> Sum1/1
  Cos/1 -> Product/2
  Product/1 -> Sum/1
  Square1/1 -> Sum1/2
  Constant/1 -> Sum/2
  Sum1/1 -> Square2/1
  Constant2/1 -> Square1/1
  Square/1 -> Gain/1
  Divide/1 -> Scope1/1, Integrator/1
  Sum/1 -> Square/1
  Square2/1 -> Divide/2
  Constant4/1 -> Square2/2
  Gain/1 -> Divide/1

== system Project_Earth_Pointing/Attitude Sensors/Earth Horizion Sensor/r_N ==
  Input1 : Inport
  Constant : Constant  Value=i
  Constant2 : Constant
  Constant3 : Constant  Value=e
  Constant4 : Constant
  Constant5 : Constant  Value=e
  Cos : Trigonometry  Operator=cos
  Cos1 : Trigonometry  Operator=cos
  Cos4 : Trigonometry  Operator=cos
  Divide : Product  Inputs=*/  RndMeth=Zero  SaturateOnIntegerOverflow=on
  Gain : Gain  Gain=a
  Normalize Vector : vrlib/Utilities/Normalize Vector  maxzero=0
  Product{,1,4..5} (4 alike) : Product
  Sin : Trigonometry
  Sin1 : Trigonometry
  Square : Math  Operator=square
  Sum : Sum  Inputs=|+-
  Sum1 : Sum  Inputs=|++
  Vector Concatenate : Concatenate  NumInputs=3
  Output : Outport
  wires:
  Input1/1 -> Cos4/1, Cos/1, Sin/1
  Constant/1 -> Sin1/1, Cos1/1
  Cos/1 -> Vector Concatenate/1
  Sin/1 -> Product1/1, Product/1
  Cos1/1 -> Product/2
  Product/1 -> Vector Concatenate/2
  Sin1/1 -> Product1/2
  Product1/1 -> Vector Concatenate/3
  Constant4/1 -> Sum1/1
  Product5/1 -> Normalize Vector/1
  Constant2/1 -> Sum/1
  Cos4/1 -> Product4/2
  Sum1/1 -> Divide/2
  Constant3/1 -> Square/1
  Product4/1 -> Sum1/2
  Square/1 -> Sum/2
  Gain/1 -> Divide/1
  Sum/1 -> Gain/1
  Constant5/1 -> Product4/1
  Divide/1 -> Product5/1
  Vector Concatenate/1 -> Product5/2
  Normalize Vector/1 -> Output/1
